simulink model "sim_lqr3tank"  (R2023a)
settings: Solver=VariableStepAuto  StartTime=0.0  StopTime=1000  RelTol=1e-3
values from neighbouring files (symbols this model uses):
  A = [-1.17e-2, 0, 1.17e-2 ... (first row only)    [lqr_3tank.m]
  B = [64.935, 0 ... (first row only)    [lqr_3tank.m]
  K = lqr(A,B,Q,R)    [lqr_3tank.m]
  r = ones(length(t), 2)    [lqr_3tank.m]
settings Model: Creator=maciel  LastModifiedBy=maciel

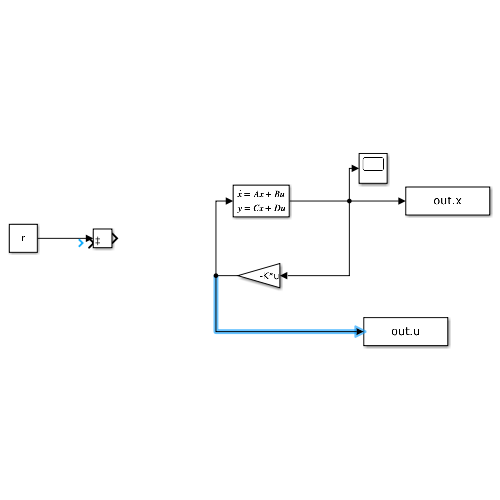
[thumbnail: Simulink's stored preview of the top-level diagram]
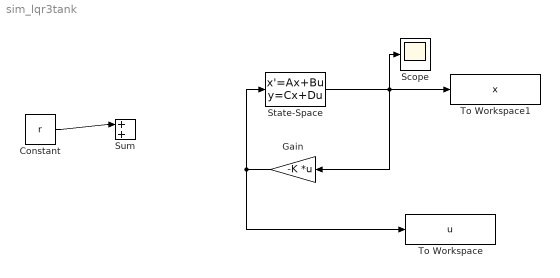
== system sim_lqr3tank ==
  Constant : Constant  Value=r  SampleTime=0.1
  Gain : Gain  Gain=-K  Multiplication=Matrix(K*u)
  Scope : Scope
  State-Space : StateSpace  A=A  B=B  C=eye(3)  D=zeros(3,2)  InitialCondition=[30; 10; 20]
  Sum : Sum  Inputs=|++
  To Workspace : ToWorkspace  VariableName=u  SaveFormat=Timeseries  SampleTime=-1
  To Workspace1 : ToWorkspace  VariableName=x  SaveFormat=Timeseries  SampleTime=-1
  wires:
  Gain/1 -> State-Space/1, To Workspace/1
  State-Space/1 -> Scope/1, To Workspace1/1, Gain/1
  Constant/1 -> Sum/1
